simulink model "hybrid_pi_control"  (R2018b)
settings: Solver=ode1  StartTime=0.0  StopTime=10  FixedStep=0.002  RelTol=1e-3  EnableMultiTasking=on
undefined symbols (not defined in the file or in its folder): HIL
libraries: quarc_library x11, simulink x1
settings Model: SimulationMode=external  ExtModeTrigDuration=10000  Creator=Student- No password  LastModifiedBy=Student-No Password
settings SolverCC: PositivePriorityOrder=on
settings DataIOCC: LimitDataPoints=on
settings OptimizationCC: LifeSpan=inf
settings DebuggingCC: AllowSymbolicDim=off  SFUnexpectedBacktrackingDiag=warning  SFNoUnconditionalDefaultTransitionDiag=warning  SFExecutionAtInitializationDiag=none
settings ModelReferenceCC: PropagateSignalLabelsOutOfModel=off
settings SFSimCC: SimUseLocalCustomCode=off
settings RTWCC: SystemTargetFile=quarc_win64.tlc  TemplateMakefile=quarc_default_tmf  Description=QUARC Win64 Target  RTWUseLocalCustomCode=off
settings CodeAppCC: StateflowObjectComments=on
settings STFCustomTargetCC: TargetPreCompLibLocation=C:\PROGRA~3\QUARC\lib\2018a\win64\release  ConcurrentExecutionCompliant=on  GRTInterface=on  SystemTargetFile=quarc_win64.tlc
settings GRTTargetCC: TargetPreCompLibLocation=C:\PROGRA~3\QUARC\lib\2018b\win64\release  TargetLangStandard=C89/C90 (ANSI)  ParMdlRefBuildCompliant=off  CompOptLevelCompliant=off  CombineOutputUpdateFcns=off  MatFileLogging=off  CPPClassGenCompliant=off  GRTInterface=on  UseToolchainInfoCompliant=off  ExtMode=on  ExtModeMexFile=quarc_comm
settings ConfigComp: CovMetricSettings=dw  CovHtmlReporting=on  CovSaveCumulativeToWorkspaceVar=on  CovSaveSingleToWorkspaceVar=on  CovExternalEMLEnable=off

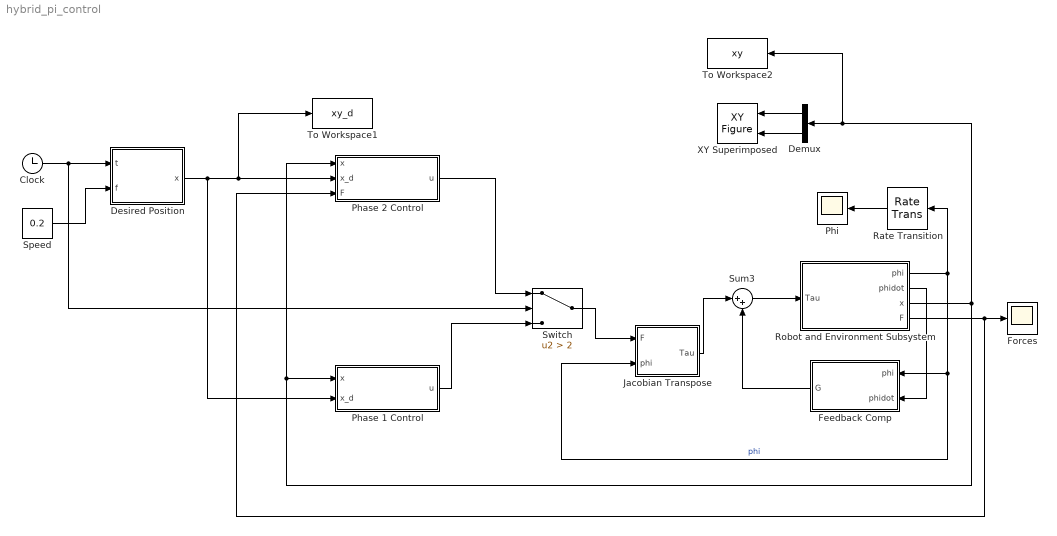
== system hybrid_pi_control ==
  Clock : Clock
  Demux : Demux  Outputs=2
  Desired Position : MATLAB Function  TreatAsAtomicUnit=on
  Feedback Comp : MATLAB Function  TreatAsAtomicUnit=on
  Forces : Scope
  Jacobian Transpose : MATLAB Function  TreatAsAtomicUnit=on
  Phase 1 Control : Subsystem
      settings: AttributesFormatString=|
      | Position Control to get from home position to benchtop
      | during t<2
  Phase 2 Control : Subsystem
      settings: AttributesFormatString=|
      | For doing force/position control on benchtop
      | during t>2
  Phi : Scope
      settings: AttributesFormatString=SampleTime =%<SampleTime>
  Rate Transition : RateTransition  OutPortSampleTimeOpt=Inherit  OutPortSampleTimeMultiple=10  OutPortSampleTime=0.05
  Robot and Environment Subsystem : Subsystem
  Speed : Constant  Value=0.2
      settings: AttributesFormatString=(strokes/sec)
  Sum3 : Sum  Inputs=|++
  Switch : Switch  Criteria=u2 > Threshold  Threshold=2
  To Workspace1 : ToWorkspace  VariableName=xy_d  SampleTime=-1
  To Workspace2 : ToWorkspace  VariableName=xy  SampleTime=-1
  XY Superimposed : quarc_library/Sinks/Figures/XY Figure  figure_mode=Use figure window  figure_tag=figure1  axes_tag=axes1  minimum_x=0.19  maximum_x=.37  minimum_y=-0.15  maximum_y=.03  buffer_size=10000  update_rate=100  initial_position="215.4         390.6         438.4         417.6"  initial_visibility=off  sample_time=-1
      settings: SourceProductName=QUARC Targets
  wires:
  Robot and Environment Subsystem/1(phi) -> Rate Transition/1, Feedback Comp/1(phi), Jacobian Transpose/2(phi)  "phi"
  Rate Transition/1 -> Phi/1
  Robot and Environment Subsystem/2(phidot) -> Feedback Comp/2(phidot)
  Feedback Comp/1(G) -> Sum3/2
  Sum3/1 -> Robot and Environment Subsystem/1(Tau)
  Jacobian Transpose/1(Tau) -> Sum3/1
  Switch/1 -> Jacobian Transpose/1(F)
  Phase 1 Control/1(u) -> Switch/3
  Clock/1 -> Desired Position/1(t), Switch/2
  Robot and Environment Subsystem/3(x) -> Phase 1 Control/1(x), Phase 2 Control/1(x), To Workspace2/1, Demux/1
  Demux/1 -> XY Superimposed/1
  Demux/2 -> XY Superimposed/2
  Robot and Environment Subsystem/4(F) -> Phase 2 Control/3(F), Forces/1
  Phase 2 Control/1(u) -> Switch/1
  Desired Position/1(x) -> To Workspace1/1, Phase 2 Control/2(x_d), Phase 1 Control/2(x_d)
  Speed/1 -> Desired Position/2(f)

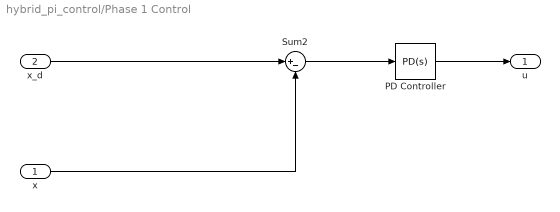
== system hybrid_pi_control/Phase 1 Control ==
  x : Inport
  x_d : Inport  Port=2
  PD Controller : simulink/Continuous/PID Controller  Controller=PD  Form=Parallel  TimeDomain=Continuous-time  SampleTime=-1  IntegratorMethod=Forward Euler  FilterMethod=Forward Euler  ControllerParametersSource=internal  P=[200;200]  I=0  D=[5;5]  UseFilter=on  N=100  TunerSelectOption=Transfer Function Based (PID Tuner App)  InitialConditionSource=internal  InitialConditionForIntegrator=0  InitialConditionForFilter=0  DifferentiatorICPrevScaledInput=0  ExternalReset=none  TrackingMode=off  Kt=1  LimitOutput=off  UpperSaturationLimit=inf  LowerSaturationLimit=-inf  LinearizeAsGain=off  AntiWindupMode=none  Kb=1  POutMin=[]  POutMax=[]  IOutMin=[]  IOutMax=[]  DOutMin=[]  DOutMax=[]  NOutMin=[]  NOutMax=[]  SumOutMin=[]  SumOutMax=[]  SaturationOutMin=[]  SaturationOutMax=[]  PParamMin=[]  PParamMax=[]  IParamMin=[]  IParamMax=[]  DParamMin=[]  DParamMax=[]  NParamMin=[]  NParamMax=[]  KbParamMin=[]  KbParamMax=[]  KtParamMin=[]  KtParamMax=[]  KbOutMin=[]  KbOutMax=[]  KtOutMin=[]  KtOutMax=[]  IntegratorOutMin=[]  IntegratorOutMax=[]  FilterOutMin=[]  FilterOutMax=[]  SumI1OutMin=[]  SumI1OutMax=[]  SumI2OutMin=[]  SumI2OutMax=[]  SumI3OutMin=[]  SumI3OutMax=[]  SumI4OutMin=[]  SumI4OutMax=[]  SumDOutMin=[]  SumDOutMax=[]  DifferentiatorOutMin=[]  DifferentiatorOutMax=[]  FilterDiffOutCoefMin=[]  FilterDiffOutCoefMax=[]  ReciprocalOutMin=[]  ReciprocalOutMax=[]  SumDenOutMin=[]  SumDenOutMax=[]  SumNumOutMin=[]  SumNumOutMax=[]  DivideOutMin=[]  DivideOutMax=[]  IntegratorContinuousStateAttributes=''  IntegratorStateMustResolveToSignalObject=off  IntegratorRTWStateStorageClass=Auto  FilterContinuousStateAttributes=''  FilterStateMustResolveToSignalObject=off  FilterRTWStateStorageClass=Auto  ParallelPVariant=InternalParameters  IdealPVariant=Disabled  IVariant=Disabled  DVariant=InternalParameters  IntegratorVariant=Disabled  SatVariant=Disabled  AWVariant=Disabled  PCopyVariant=Disabled  TRVariant=Disabled  FdbkBlocksVariant=Forward  IdealPFdbkVariant=Disabled  SatFdbkVariant=Disabled  DerivativeFilterVariant=ContFilter  NVariant=InternalParameters  NCopyVariant=Disabled  FilterICVariant=InternalICsFilter  IntegratorICVariant=Disabled  ExternalResetVariant=Disabled  TRSumVariant=Passthrough  SumFdbkVariant=Disabled  SumVariant=Sum_PD
      settings: AttributesFormatString='PGain='%<P>\n'DGain='%<D>
  Sum2 : Sum  Inputs=|+-
  u : Outport
  wires:
  Sum2/1 -> PD Controller/1
  x/1 -> Sum2/2
  PD Controller/1 -> u/1
  x_d/1 -> Sum2/1

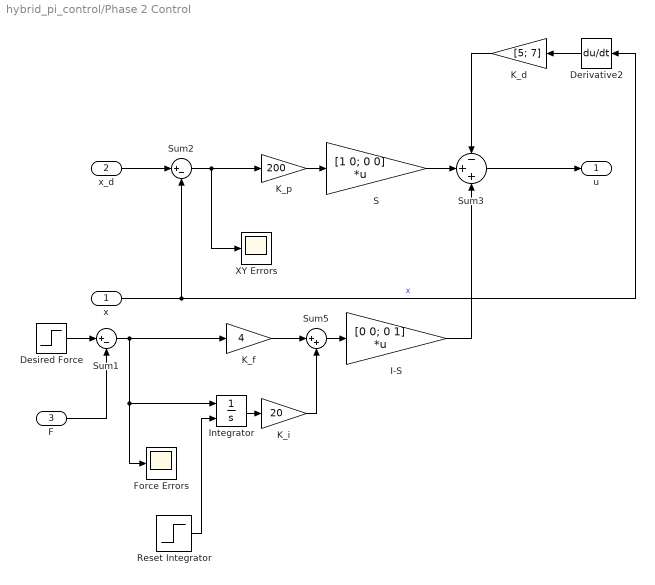
== system hybrid_pi_control/Phase 2 Control ==
  x : Inport
  x_d : Inport  Port=2
  F : Inport  Port=3
  " K_p" : Gain  Gain=200
  Derivative2 : Derivative
  Desired Force : Step  Time=2  After=[0;-1]  SampleTime=0
      settings: AttributesFormatString=|
      | F=%<After>
      | @time>%<Time>
  Force Errors : Scope
  I-S : Gain  Gain=[0 0; 0 1]  Multiplication=Matrix(K*u)
  Integrator : Integrator  ExternalReset=rising
  K_d : Gain  Gain=[5; 7]
  K_f : Gain  Gain=4
  K_i : Gain  Gain=20
  Reset Integrator : Step  Time=2  SampleTime=0
      settings: AttributesFormatString=@time=%<Time>
  S : Gain  Gain=[1 0; 0 0]  Multiplication=Matrix(K*u)
  Sum1 : Sum  Inputs=|+-
  Sum2 : Sum  Inputs=|+-
  Sum3 : Sum  Inputs=-++
  Sum5 : Sum  Inputs=|++
  XY Errors : Scope
  u : Outport
  wires:
  Sum2/1 -> " K_p"/1, XY Errors/1
  Sum3/1 -> u/1
  Desired Force/1 -> Sum1/1
  x_d/1 -> Sum2/1
  F/1 -> Sum1/2
  Sum1/1 -> K_f/1, Force Errors/1, Integrator/1
  Integrator/1 -> K_i/1
  Reset Integrator/1 -> Integrator/2
  S/1 -> Sum3/2
  " K_p"/1 -> S/1
  K_d/1 -> Sum3/1
  Derivative2/1 -> K_d/1
  x/1 -> Derivative2/1, Sum2/2  "x"
  K_i/1 -> Sum5/2
  K_f/1 -> Sum5/1
  Sum5/1 -> I-S/1
  I-S/1 -> Sum3/3

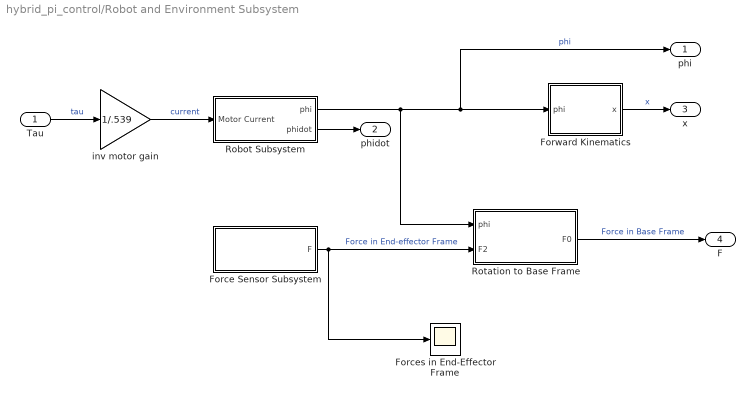
== system hybrid_pi_control/Robot and Environment Subsystem ==
  Tau : Inport
  Force Sensor Subsystem : Subsystem
  Forces in End-Effector Frame : Scope
  Forward Kinematics : MATLAB Function  TreatAsAtomicUnit=on
  Robot Subsystem : Subsystem
  Rotation to Base Frame : MATLAB Function  TreatAsAtomicUnit=on
  inv motor gain : Gain  Gain=1/.539
  phi : Outport
  phidot : Outport  Port=2
  x : Outport  Port=3
  F : Outport  Port=4
  wires:
  Robot Subsystem/1(phi) -> Rotation to Base Frame/1(phi), phi/1, Forward Kinematics/1(phi)  "phi"
  Forward Kinematics/1(x) -> x/1  "x"
  inv motor gain/1 -> Robot Subsystem/1(Motor Current)  "current"
  Tau/1 -> inv motor gain/1  "tau"
  Robot Subsystem/2(phidot) -> phidot/1
  Force Sensor Subsystem/1(F) -> Forces in End-Effector Frame/1, Rotation to Base Frame/2(F2)  "Force in End-effector Frame"
  Rotation to Base Frame/1(F0) -> F/1  "Force in Base Frame"

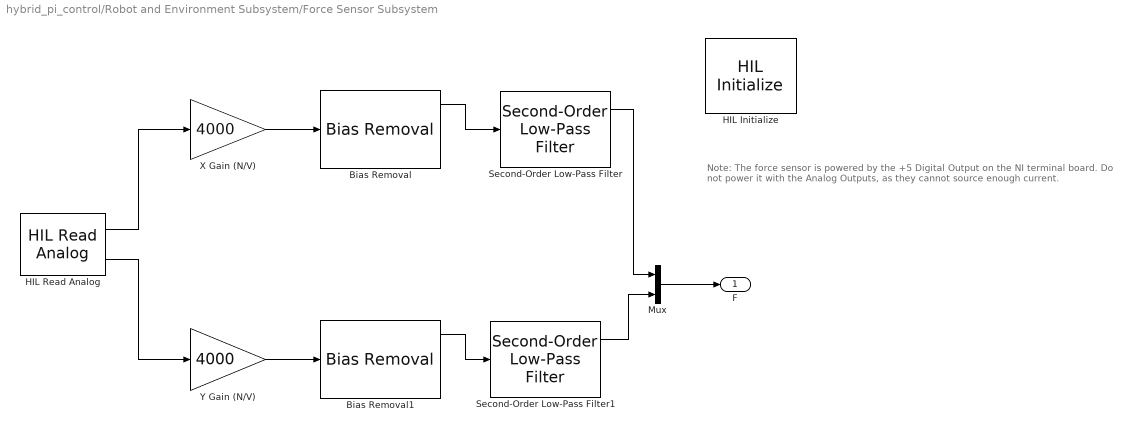
== system hybrid_pi_control/Robot and Environment Subsystem/Force Sensor Subsystem ==
  note: Note: The force sensor is powered by the +5 Digital Output on the NI terminal board.
      | Do not power it with the Analog Outputs, as they cannot source enough current.
  Bias Removal : quarc_library/Discrete/Bias Removal  start_time=0.1  end_time=0.5  switch_id=0  sample_time=qc_get_step_size
      settings: SourceProductName=QUARC Targets
  Bias Removal1 : quarc_library/Discrete/Bias Removal  start_time=0.1  end_time=0.5  switch_id=0  sample_time=qc_get_step_size
      settings: SourceProductName=QUARC Targets
  HIL Initialize : quarc_library/Data Acquisition/Generic/Configuration/HIL Initialize  Priority=-99  object_name=NI  board_type=ni_pci_6014  board_number=0  board_options=terminal_board=e_series  exclusive=off  active=off  hardware_clocks=[]  clock_modes=[]  initial_clock_frequencies=[]  set_clock_params_at_start=off  set_clock_params_at_switch_in=off  set_clock_frequencies_at_start=off  set_clock_frequencies_at_switch_in=off  analog_input_channels=[]  analog_input_configurations=[]  analog_input_maximums=10  analog_input_minimums=-10  set_analog_input_params_at_start=on  set_analog_input_params_at_switch_in=off  analog_output_channels=[0]  analog_output_maximums=10  analog_output_minimums=-10  initial_analog_outputs=[0]  final_analog_outputs=[0]  watchdog_analog_outputs=[]  set_analog_output_params_at_start=off  set_analog_output_params_at_switch_in=off  set_analog_outputs_at_start=on  set_analog_outputs_at_switch_in=off  set_analog_outputs_at_terminate=on  set_analog_outputs_at_switch_out=off  set_analog_outputs_on_watchdog=off  digital_input_channels=[]  digital_output_channels=[]  digital_output_configuration=[]  initial_digital_outputs=[1]  final_digital_outputs=[1]  watchdog_digital_outputs=[]  set_digital_output_params_at_start=off  set_digital_output_params_at_switch_in=off  set_digital_outputs_at_start=on  set_digital_outputs_at_switch_in=off  set_digital_outputs_at_terminate=on  set_digital_outputs_at_switch_out=off  set_digital_outputs_on_watchdog=off  encoder_channels=[]  quadrature=[0]  encoder_filter_frequency=[]  initial_encoder_counts=[0]  set_encoder_params_at_start=on  set_encoder_params_at_switch_in=off  set_encoder_counts_at_start=on  set_encoder_counts_at_switch_in=off  pwm_channels=[]  pwm_modes=[0]  pwm_frequency=20e6/4096  pwm_configuration=[]  pwm_alignment=[]  pwm_polarity=[]  pwm_leading_deadband=[]  pwm_trailing_deadband=[]  initial_pwm_outputs=[0]  final_pwm_outputs=[0]  watchdog_pwm_outputs=[]  set_pwm_params_at_start=on  set_pwm_params_at_switch_in=off  set_pwm_outputs_at_start=on  set_pwm_outputs_at_switch_in=off  set_pwm_outputs_at_terminate=on  set_pwm_outputs_at_switch_out=off  set_pwm_outputs_on_watchdog=off  other_output_channels=[]  initial_other_outputs=[]  final_other_outputs=[]  watchdog_other_outputs=[]  set_other_outputs_at_start=off  set_other_outputs_at_switch_in=off  set_other_outputs_at_terminate=off  set_other_outputs_at_switch_out=off  set_other_outputs_on_watchdog=off
  HIL Read Analog : quarc_library/Data Acquisition/Generic/Immediate I//O/HIL Read Analog  object_name=NI  channels=[0 1]  sample_time=qc_get_step_size  active=on  vector_output=off
  Mux : Mux  Inputs=2
  Second-Order Low-Pass Filter : quarc_library/Continuous/Second-Order Low-Pass Filter  params_source=Internal (dialog parameters)  input_width=10  input_zeta=1  input_init=0
  Second-Order Low-Pass Filter1 : quarc_library/Continuous/Second-Order Low-Pass Filter  params_source=Internal (dialog parameters)  input_width=10  input_zeta=1  input_init=0
  X Gain (N/V) : Gain  Gain=4000
  Y Gain (N/V) : Gain  Gain=4000
  F : Outport
  wires:
  HIL Read Analog/1 -> X Gain (N/V)/1
  X Gain (N/V)/1 -> Bias Removal/1
  HIL Read Analog/2 -> Y Gain (N/V)/1
  Y Gain (N/V)/1 -> Bias Removal1/1
  Mux/1 -> F/1
  Bias Removal/1 -> Second-Order Low-Pass Filter/1
  Bias Removal1/1 -> Second-Order Low-Pass Filter1/1
  Second-Order Low-Pass Filter/1 -> Mux/1
  Second-Order Low-Pass Filter1/1 -> Mux/2

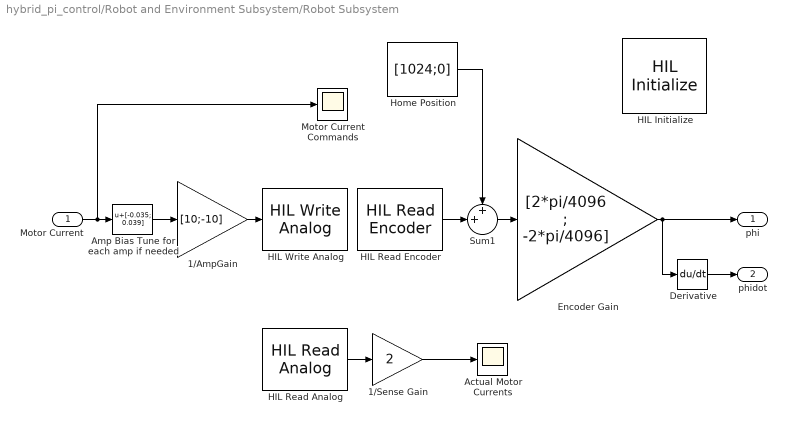
== system hybrid_pi_control/Robot and Environment Subsystem/Robot Subsystem ==
  Motor Current : Inport
  1/AmpGain : Gain  Gain=[10;-10]
  1/Sense Gain : Gain  Gain=2
  Actual Motor Currents : Scope
  Amp Bias Tune for each amp if needed : Bias  Bias=[-0.035; 0.039]
  Derivative : Derivative
  Encoder Gain : Gain  Gain=[2*pi/4096 ; -2*pi/4096]
  HIL Initialize : quarc_library/Data Acquisition/Generic/Configuration/HIL Initialize  object_name=HIL-1  board_type=q8_usb  board_number=0  board_options=update_rate=normal  exclusive=off  active=off  hardware_clocks=[0:2]  clock_modes=[]  initial_clock_frequencies=[]  set_clock_params_at_start=off  set_clock_params_at_switch_in=off  set_clock_frequencies_at_start=off  set_clock_frequencies_at_switch_in=off  analog_input_channels=[0:7]  analog_input_configurations=[]  analog_input_maximums=10  analog_input_minimums=-10  set_analog_input_params_at_start=on  set_analog_input_params_at_switch_in=off  analog_output_channels=[0:7]  analog_output_maximums=10  analog_output_minimums=-10  initial_analog_outputs=[0]  final_analog_outputs=[0]  watchdog_analog_outputs=0  set_analog_output_params_at_start=on  set_analog_output_params_at_switch_in=off  set_analog_outputs_at_start=on  set_analog_outputs_at_switch_in=off  set_analog_outputs_at_terminate=on  set_analog_outputs_at_switch_out=off  set_analog_outputs_on_watchdog=off  digital_input_channels=[]  digital_output_channels=[]  digital_output_configuration=[]  initial_digital_outputs=[1]  final_digital_outputs=[1]  watchdog_digital_outputs=[1]  set_digital_output_params_at_start=off  set_digital_output_params_at_switch_in=off  set_digital_outputs_at_start=on  set_digital_outputs_at_switch_in=off  set_digital_outputs_at_terminate=on  set_digital_outputs_at_switch_out=off  set_digital_outputs_on_watchdog=off  encoder_channels=[0:7]  quadrature=[4]  encoder_filter_frequency=[]  initial_encoder_counts=[0]  set_encoder_params_at_start=on  set_encoder_params_at_switch_in=off  set_encoder_counts_at_start=on  set_encoder_counts_at_switch_in=off  pwm_channels=[0:7]  pwm_modes=0  pwm_frequency=99.532799999999995e6/4095  pwm_configuration=[0]  pwm_alignment=[0]  pwm_polarity=[1]  pwm_leading_deadband=[0]  pwm_trailing_deadband=[0]  initial_pwm_outputs=[0]  final_pwm_outputs=[0]  watchdog_pwm_outputs=[0]  set_pwm_params_at_start=on  set_pwm_params_at_switch_in=off  set_pwm_outputs_at_start=on  set_pwm_outputs_at_switch_in=off  set_pwm_outputs_at_terminate=on  set_pwm_outputs_at_switch_out=off  set_pwm_outputs_on_watchdog=off  other_output_channels=[]  initial_other_outputs=[]  final_other_outputs=[]  watchdog_other_outputs=[]  set_other_outputs_at_start=off  set_other_outputs_at_switch_in=off  set_other_outputs_at_terminate=off  set_other_outputs_at_switch_out=off  set_other_outputs_on_watchdog=off
  HIL Read Analog : quarc_library/Data Acquisition/Generic/Immediate I//O/HIL Read Analog  object_name=HIL-1  channels=[0;1]  sample_time=qc_get_step_size  active=on  vector_output=on
  HIL Read Encoder : quarc_library/Data Acquisition/Generic/Immediate I//O/HIL Read Encoder  object_name=HIL-1  channels=[0:1]  sample_time=qc_get_step_size  active=on  vector_output=on  data_type_mode=Inherit via back propagation  data_type=double
  HIL Write Analog : quarc_library/Data Acquisition/Generic/Immediate I//O/HIL Write Analog  object_name=HIL-1  channels=[0:1]  sample_time=-1  active=off  vector_input=on
  Home Position : Constant  Value=[1024;0]  VectorParams1D=off
  Motor Current Commands : Scope
  Sum1 : Sum  Inputs=++|
  phi : Outport
  phidot : Outport  Port=2
  wires:
  1/AmpGain/1 -> HIL Write Analog/1
  Encoder Gain/1 -> phi/1, Derivative/1
  Derivative/1 -> phidot/1
  1/Sense Gain/1 -> Actual Motor Currents/1
  HIL Read Analog/1 -> 1/Sense Gain/1
  Motor Current/1 -> Amp Bias Tune for each amp if needed/1, Motor Current Commands/1
  Amp Bias Tune for each amp if needed/1 -> 1/AmpGain/1
  Home Position/1 -> Sum1/1
  HIL Read Encoder/1 -> Sum1/2
  Sum1/1 -> Encoder Gain/1

== matlab function hybrid_pi_control/Desired Position ==
  settings: fimath=|
      | fimath(...
      | 'RoundMode', 'floor',...
      | 'OverflowMode', 'wrap',...
      | 'ProductMode', 'KeepLSB', 'ProductWordLength', 32,...
      | 'SumMode', 'KeepLSB', 'SumWordLength', 32,...
      | 'CastBeforeSum', false)
  data: x output; t input; f input
function x = fcn(t,f)
% This block supports an embeddable subset of the MATLAB language.
% See the help menu for details. 
x = [0;0];

h = -0.06; % wall height
L = 0.07; % force sensor length

if t<2 % Phase 1 will be in control during first 2 seconds to move from home position to point on benchtop
        x(1) = 0.15 + L + 0.0375*(1 - cos(pi*t/2));
        x(2) = 0.15 - (0.15-h)/2*(1 - cos(pi*t/2));
elseif t<2.5  % Now Phase 2 accelerates into stroking trajectory
    x(1) = 0.075*cos(2*pi*f*(t-2)^2) + 0.15 + L;
    x(2) = h;
else  % Phase 2 continues stroking trajectory along benchtop
    x(1) = 0.075*cos(2*pi*f*(t-2.25)) + 0.15 + L;
    x(2) = h;
end

== matlab function hybrid_pi_control/Feedback Comp ==
  settings: fimath=|
      | fimath(...
      | 'RoundMode', 'floor',...
      | 'OverflowMode', 'wrap',...
      | 'ProductMode', 'KeepLSB', 'ProductWordLength', 32,...
      | 'SumMode', 'KeepLSB', 'SumWordLength', 32,...
      | 'CastBeforeSum', false)
  data: G output; phi input; phidot input
function G = fcn(phi, phidot)
% This block supports an embeddable subset of the MATLAB language.
% See the help menu for details. 

a1 = 0.15;  % link 1 length
a2 = 0.15;  % link 2 length
m1 = 0.092;  % link 1 mass  
m2 = 0.077+0.03; % link 2 mass
r01 = 0.062; % link 1 center of mass
r12 = 0.036+0.04; % link 2 COM

g = 9.8; % gravitational constant

G1 = (r01*m1+a1*m2)*g*cos(phi(1));
G2 = r12*m2*g*cos(phi(2));

G = [G1;G2]; % gravity torques

== matlab function hybrid_pi_control/Jacobian Transpose ==
  settings: fimath=|
      | fimath(...
      | 'RoundMode', 'floor',...
      | 'OverflowMode', 'wrap',...
      | 'ProductMode', 'KeepLSB', 'ProductWordLength', 32,...
      | 'SumMode', 'KeepLSB', 'SumWordLength', 32,...
      | 'CastBeforeSum', false)
  data: F input; Tau output; phi input
function Tau = fcn(F,phi)
% This block supports an embeddable subset of the MATLAB language.
% See the help menu for details. 
a1=0.15;
a2=0.15;

J11 = -a1*sin(phi(1));
J12 = -a2*sin(phi(2));
J21 = a1*cos(phi(1));
J22 = a2*cos(phi(2));

J = [J11 J12; J21 J22];

Tau = J'*F;

== matlab function hybrid_pi_control/Robot and Environment Subsystem/Forward Kinematics ==
  settings: fimath=|
      | fimath(...
      | 'RoundMode', 'floor',...
      | 'OverflowMode', 'wrap',...
      | 'ProductMode', 'KeepLSB', 'ProductWordLength', 32,...
      | 'SumMode', 'KeepLSB', 'SumWordLength', 32,...
      | 'CastBeforeSum', false)
  data: x output; phi input
function x = fcn(phi)
% This block supports an embeddable subset of the MATLAB language.
% See the help menu for details. 

a1=0.15;
a2=0.15+0.07; %modified to include length of force sensor
x = [0;0];
x(1) = a1*cos(phi(1))+a2*cos(phi(2));
x(2) = a1*sin(phi(1))+a2*sin(phi(2));

== matlab function hybrid_pi_control/Robot and Environment Subsystem/Rotation to Base Frame ==
  settings: fimath=|
      | fimath(...
      | 'RoundMode', 'floor',...
      | 'OverflowMode', 'wrap',...
      | 'ProductMode', 'KeepLSB', 'ProductWordLength', 32,...
      | 'SumMode', 'KeepLSB', 'SumWordLength', 32,...
      | 'CastBeforeSum', false)
  data: phi input; F0 output; F2 input
function F0 = fcn(phi,F2)
% This block supports an embeddable subset of the MATLAB language.
% See the help menu for details. 



R = [cos(phi(2)) , -sin(phi(2));
     sin(phi(2)) , cos(phi(2))];


F0 = R*F2;
